simulink model "Lab03_Q2_Sim"  (R2024a)
settings: Solver=VariableStepAuto  StartTime=0.0  StopTime=600  RelTol=1e-3
values from neighbouring files (symbols this model uses):
  C_T = H'    [Lab03_Q2.m]    (also in Lab03_Q2_Data.mat = [0 1])
  G_dc_inv_db = 1 / dcgain(sys_db)    [Lab03_Q2.m]    (also in Lab03_Q2_Data.mat = 16.2558130405)
  G_dc_inv_ndb = 1 / dcgain(sys_ndb)    [Lab03_Q2.m]    (also in Lab03_Q2_Data.mat = 0.104037203459)
  G_T = G'    [Lab03_Q2.m]    (also in Lab03_Q2_Data.mat = [0  -0.289176820335; 1  1.26502539796])
  H_T = C'    [Lab03_Q2.m]    (also in Lab03_Q2_Data.mat = [0.0385501764157 0.0229662791138])
  L_db = acker(G_T, H_T, desired_poles_db)    [Lab03_Q2.m]    (also in Lab03_Q2_Data.mat = [20.085372175 21.367447239])
  L_ndb = acker(G_T, H_T, desired_poles_ndb)    [Lab03_Q2.m]    (also in Lab03_Q2_Data.mat = [-12.6739055175 -3.76174599436])
libraries: simulink x1
settings Model: Creator=24246  LastModifiedBy=24246
settings DataIOCC: ReturnWorkspaceOutputs=off

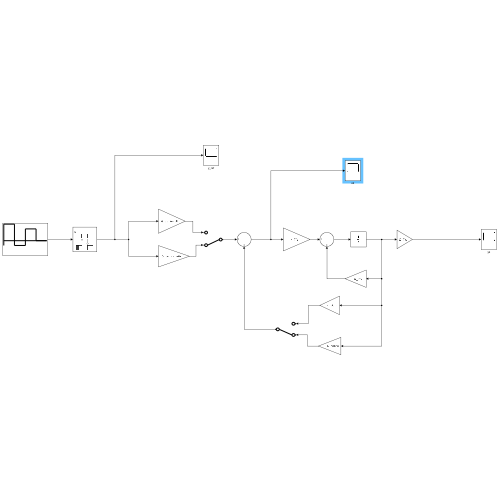
[thumbnail: Simulink's stored preview of the top-level diagram]
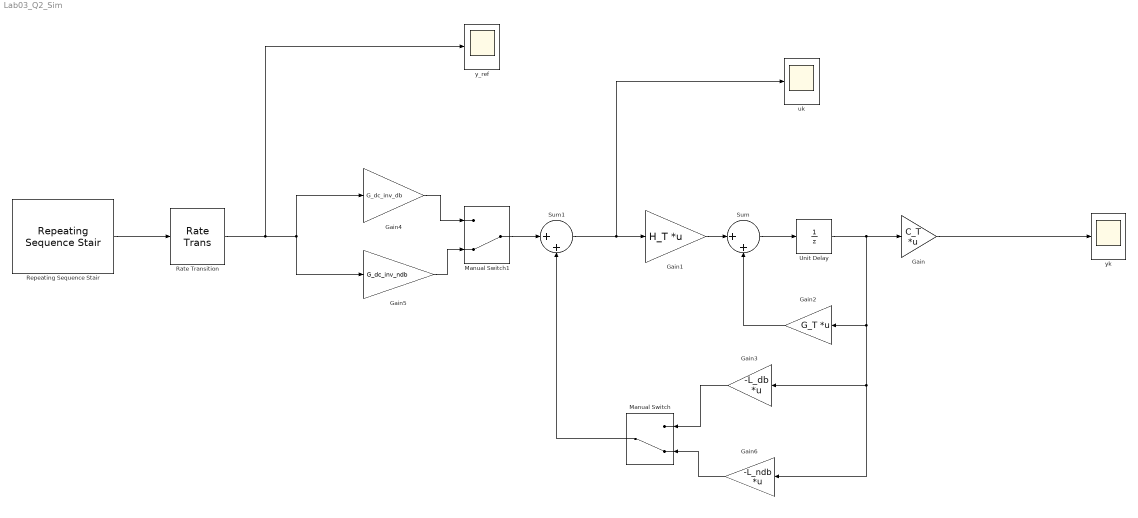
== system Lab03_Q2_Sim ==
  Gain : Gain  Gain=C_T  Multiplication=Matrix(K*u)
  Gain1 : Gain  Gain=H_T  Multiplication=Matrix(K*u)
  Gain2 : Gain  Gain=G_T  Multiplication=Matrix(K*u)
  Gain3 : Gain  Gain=-L_db  Multiplication=Matrix(K*u)
  Gain4 : Gain  Gain=G_dc_inv_db
  Gain5 : Gain  Gain=G_dc_inv_ndb
  Gain6 : Gain  Gain=-L_ndb  Multiplication=Matrix(K*u)
  Manual Switch : ManualSwitch  CurrentSetting=0
  Manual Switch1 : ManualSwitch  CurrentSetting=0
  Rate Transition : RateTransition  OutPortSampleTime=0.75
  Repeating Sequence Stair : simulink/Sources/Repeating Sequence Stair  OutValues=[0.7 -0.2 0.5 0]'  tsamp=105  OutMin=[]  OutMax=[]  OutDataTypeStr=double  OutputDataTypeScalingMode=double  OutDataType=fixdt(0,8)  ConRadixGroup=Best Precision: Vector-wise  OutScaling=2^-12
  Sum : Sum  Inputs=|++
  Sum1 : Sum  Inputs=|++
  Unit Delay : UnitDelay  InitialCondition=[0 0]  SampleTime=0.75  HasFrameUpgradeWarning=on
  uk : Scope
  y_ref : Scope
  yk : Scope
  wires:
  Manual Switch1/1 -> Sum1/1
  Gain5/1 -> Manual Switch1/2
  Gain3/1 -> Manual Switch/1
  Gain6/1 -> Manual Switch/2
  Manual Switch/1 -> Sum1/2
  Gain4/1 -> Manual Switch1/1
  Unit Delay/1 -> Gain6/1, Gain3/1, Gain2/1, Gain/1
  Repeating Sequence Stair/1 -> Rate Transition/1
  Sum1/1 -> uk/1, Gain1/1
  Sum/1 -> Unit Delay/1
  Gain1/1 -> Sum/1
  Gain2/1 -> Sum/2
  Rate Transition/1 -> y_ref/1, Gain4/1, Gain5/1
  Gain/1 -> yk/1
